simulink model "a1"  (R2019b)
settings: Solver=VariableStepAuto  StartTime=0.0  StopTime=20  RelTol=1e-3
undefined symbols (not defined in the file or in its folder): drawArm
settings Model: PacingRate=11  Creator=Akhil Jarodia  LastModifiedBy=Akhil Jarodia

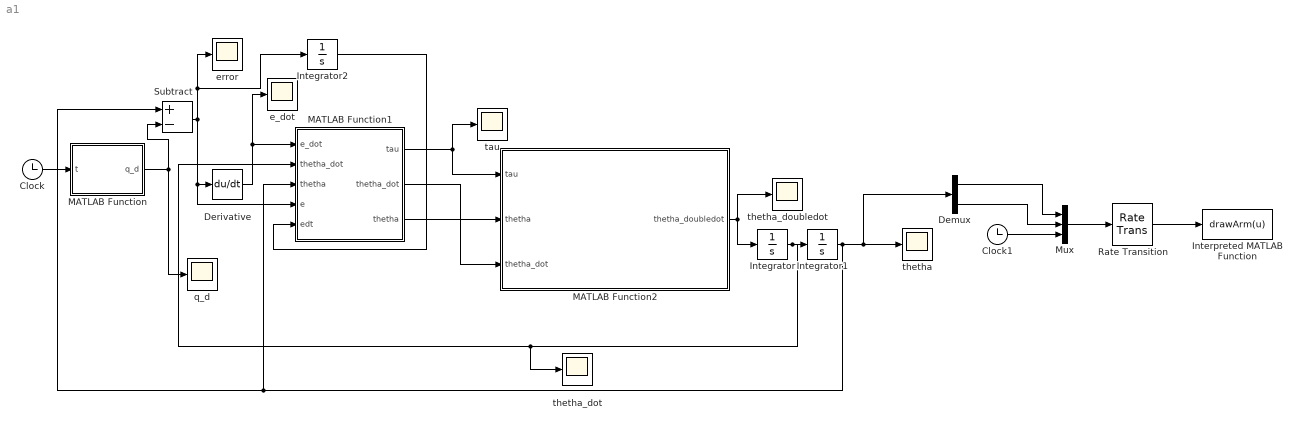
== system a1 ==
  Clock : Clock
      settings: Decimation=50
  Clock1 : Clock
      settings: Decimation=50
  Demux : Demux  Outputs=2
  Derivative : Derivative
  Integrator : Integrator  InitialCondition=[0;0]
  Integrator1 : Integrator  InitialCondition=[0;0]
  Integrator2 : Integrator  InitialCondition=[0;0]
  Interpreted MATLAB Function : MATLABFcn  MATLABFcn=drawArm(u)  OutputDimensions=0
  MATLAB Function : MATLAB Function  TreatAsAtomicUnit=on
  MATLAB Function1 : MATLAB Function  TreatAsAtomicUnit=on
  MATLAB Function2 : MATLAB Function  TreatAsAtomicUnit=on
  Mux : Mux  Inputs=3
  Rate Transition : RateTransition
  Subtract : Sum  Inputs=+-
  e_dot : Scope
  error : Scope
  q_d : Scope
  tau : Scope
  thetha : Scope
  "thetha_dot " : Scope
  thetha_doubledot : Scope
  wires:
  Clock/1 -> MATLAB Function/1(t)
  Derivative/1 -> e_dot/1, MATLAB Function1/1(e_dot)
  MATLAB Function1/1(tau) -> MATLAB Function2/1(tau), tau/1
  MATLAB Function2/1(thetha_doubledot) -> Integrator/1, thetha_doubledot/1
  Integrator/1 -> MATLAB Function1/2("thetha_dot "), "thetha_dot "/1, Integrator1/1
  Integrator1/1 -> Subtract/1, MATLAB Function1/3("thetha "), Demux/1, thetha/1
  MATLAB Function/1(q_d) -> Subtract/2, q_d/1
  Subtract/1 -> MATLAB Function1/4(e), Derivative/1, Integrator2/1, error/1
  MATLAB Function1/2(thetha_dot) -> MATLAB Function2/3(thetha_dot)
  MATLAB Function1/3(thetha) -> MATLAB Function2/2(thetha)
  Rate Transition/1 -> Interpreted MATLAB Function/1
  Mux/1 -> Rate Transition/1
  Demux/1 -> Mux/1
  Clock1/1 -> Mux/3
  Demux/2 -> Mux/2
  Integrator2/1 -> MATLAB Function1/5(edt)

== matlab function a1/MATLAB Function1 ==
  data: e_dot input; thetha_dot input; thetha input; e input; tau output; thetha_dot output; thetha output; edt input
function [tau,thetha_dot,thetha]= controller(e_dot,thetha_dot,thetha,e, edt)

tau = -5.*e-5.*e_dot;
thetha_dot=thetha_dot;
thetha=thetha;

== matlab function a1/MATLAB Function ==
  data: q_d output; t input
function q_d = angle(t)


% q_d = [pi/3 ;pi/4];

q_d=[sin(t); cos(t)];

== matlab function a1/MATLAB Function2 ==
  data: tau input; thetha_doubledot output; thetha input; thetha_dot input
function thetha_doubledot = fcn(tau,thetha,thetha_dot)
m1=1;g=9.8;
m2=1;
a1=1;a2=1;
t1=thetha(1);t2=thetha(2);
t1_dot=thetha_dot(1);t2_dot=thetha_dot(2);


M=[(m1*a1*a1 + m2*(a1*a1 + 2*a1*a2*cos(t2)+a2*a2)), (m2*(a1*a2*cos(t2)+ a2*a2));
    (m2*(a1*a2*cos(t2)+ a2*a2)) ,m2*a2*a2];

V=[(-m2*a1*a2*sin(t2)*(2*t1_dot*t2_dot + t2_dot*t2_dot ));
    m2*a1*a2*t1_dot*t1_dot*sin(t2)];
G=[((m1+m2)*a1*g*cos(t1) + m2*g*a2*cos(t1+t2));
    m2*g*a2*cos(t1+t2)];


thetha_doubledot=inv(M)*(tau-(V)-G);
